simulink model "double_SDM_CoSim"  (R2023b)
settings: Solver=VariableStepAuto  StartTime=0.0  StopTime=10.0  RelTol=1e-3
values from neighbouring files (symbols this model uses):
  Ts = 0.001    [main.m]
undefined symbols (not defined in the file or in its folder): CEcosimulation, CoSimulate1
libraries: cstblocks x4, instrumentlib x2
settings Model: Creator=Aleksandr Prokhorov  LastModifiedBy=Aleksandr Prokhorov

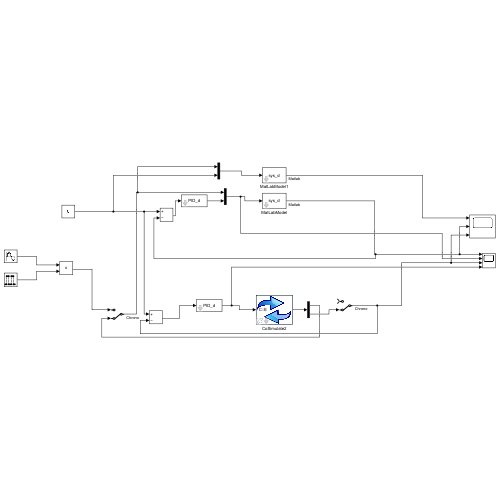
[thumbnail: Simulink's stored preview of the top-level diagram]
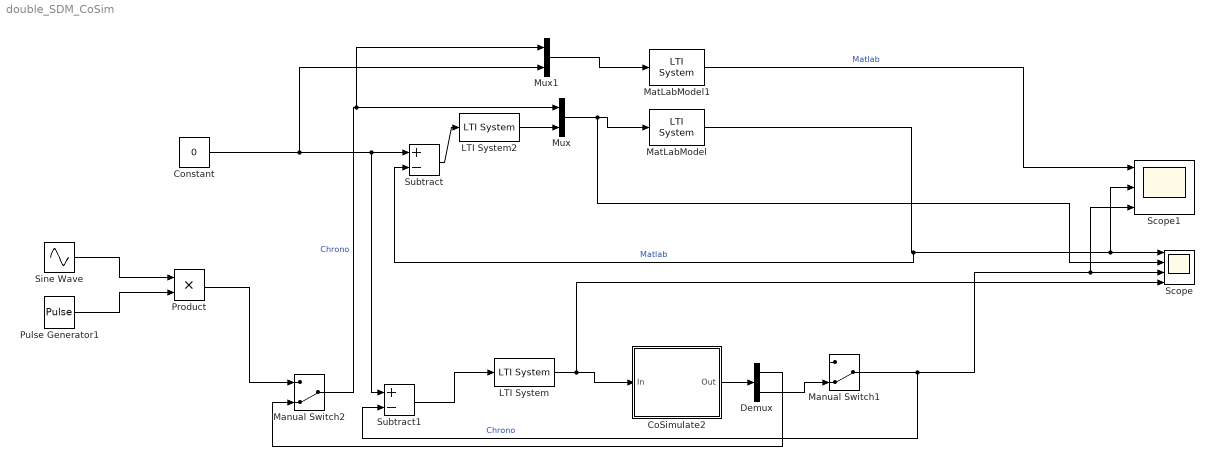
== system double_SDM_CoSim ==
  CoSimulate2 : Subsystem  Description=|  Priority=100  AncestorBlock=CEcosimulation/CoSimulate1  mask{com_step=Ts, tcp_data_size=2, host_name=localhost, tcp_port=50009, tcp_timeout=15}
      | This block can be used to exchange data with Chrono::Engine.                                                                                      
      | A Chrono::Engine program with a running ChCosimulation inferface must be started, it will work as a server; then the Simulink program must be run.
      | Note! check that the dimensions of the exchanged vectors do match!
      mask prompts: com_step "Communication step size"; tcp_data_size "N. of scalars received from C::E (as block output)"; host_name "TCP host name (ex. 'localhost', or 'www.myhost.com')"; tcp_port "TCP port (ex. 50007)"; tcp_timeout "TCP timeout (seconds)"
      mask init:
      | block_receive = [gcb, '/TCP Receive'];
      | set_param(block_receive, 'SampleTime', num2str(com_step));
      | set_param(block_receive, 'Host', host_name);
      | set_param(block_receive, 'Port', num2str(tcp_port));
      | set_param(block_receive, 'DataSize', num2str(tcp_data_size+1));
      | set_param(block_receive, 'Timeout', num2str(tcp_timeout));
      | block_send = [gcb, '/TCP Send'];
      | set_param(block_send, 'Host', host_name);
      | set_param(block_send, 'Port', num2str(tcp_port));
      mask Display:
      | image(imread('block_logo.png'))
      | disp('C::E                   ')
  Constant : Constant  Value=0  SampleTime=Ts
  Demux : Demux  Outputs=2
  LTI System : cstblocks/LTI System  sys=PID_d  IC=[]  PadeOrder=0
  LTI System2 : cstblocks/LTI System  sys=PID_d  IC=[]  PadeOrder=0
  Manual Switch1 : ManualSwitch  CurrentSetting=0
  Manual Switch2 : ManualSwitch  CurrentSetting=0
  MatLabModel : cstblocks/LTI System  sys=sys_d  IC=[]  PadeOrder=0
  MatLabModel1 : cstblocks/LTI System  sys=sys_d  IC=[]  PadeOrder=0
  Mux : Mux  Inputs=2
  Mux1 : Mux  Inputs=2
  Product : Product
  Pulse Generator1 : DiscretePulseGenerator  Period=10/Ts  PulseWidth=0.05/Ts  PhaseDelay=1/Ts  SampleTime=Ts
  Scope : Scope  NumInputPorts=4
  Scope1 : Scope  NumInputPorts=3
  Sine Wave : Sin  Frequency=50  Phase=0.35  SampleTime=Ts
  Subtract : Sum  Inputs=+-
  Subtract1 : Sum  Inputs=+-
  wires:
  Pulse Generator1/1 -> Product/2
  Manual Switch1/1 -> Subtract1/2, Scope/3, Scope1/3  "Chrono"
  MatLabModel/1 -> Subtract/2, Scope/1, Scope1/2  "Matlab"
  Sine Wave/1 -> Product/1
  Mux/1 -> Scope/2, MatLabModel/1
  CoSimulate2/1(Out) -> Demux/1
  Demux/2 -> Manual Switch1/2
  Product/1 -> Manual Switch2/1
  Demux/1 -> Manual Switch2/2
  Manual Switch2/1 -> Mux1/1, Mux/1  "Chrono"
  Subtract1/1 -> LTI System/1
  Subtract/1 -> LTI System2/1
  LTI System/1 -> Scope/4, CoSimulate2/1(In)
  MatLabModel1/1 -> Scope1/1  "Matlab"
  Mux1/1 -> MatLabModel1/1
  Constant/1 -> Mux1/2, Subtract/1, Subtract1/1
  LTI System2/1 -> Mux/2

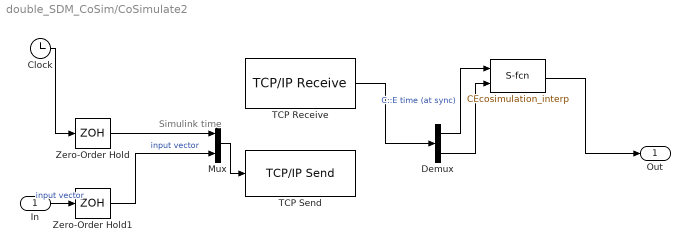
== system double_SDM_CoSim/CoSimulate2 ==
  note: Simulink time
  In : Inport
  " " : M-S-Function  FunctionName=CEcosimulation_interp
  Clock : Clock
  Demux : Demux  Outputs=[1 -1]
  Mux : Mux  Inputs=2
  TCP Receive : instrumentlib/TCP//IP Receive  Priority=1  Host=localhost  Port=50009  DataSize=3  DataType=double  ASCIIFormatting=%f  Terminator=LF  CustomTerminator=10  ByteOrder=little-endian  EnableBlockingMode=on  Timeout=15  SampleTime=0.001  SimulateUsing=Interpreted execution
  TCP Send : instrumentlib/TCP//IP Send  Priority=2  Host=localhost  Port=50009  ByteOrder=little-endian  EnableBlockingMode=on  Timeout=10  TransferDelay=on  SimulateUsing=Interpreted execution
  Zero-Order Hold : ZeroOrderHold  Priority=0  SampleTime=com_step
  Zero-Order Hold1 : ZeroOrderHold  Priority=0  SampleTime=com_step
  Out : Outport
  wires:
  " "/1 -> Out/1
  Demux/2 -> " "/2
  Demux/1 -> " "/1  "C::E time (at sync)"
  Zero-Order Hold/1 -> Mux/1
  Zero-Order Hold1/1 -> Mux/2  "input vector"
  Mux/1 -> TCP Send/1
  Clock/1 -> Zero-Order Hold/1
  In/1 -> Zero-Order Hold1/1  "input vector"
  TCP Receive/1 -> Demux/1
